simulink model "bai27_Simulink"  (R2016a)
settings: Solver=VariableStepAuto  StartTime=0.0  StopTime=10.0  RelTol=1e-3
settings Model: Creator=HP  LastModifiedBy=HP

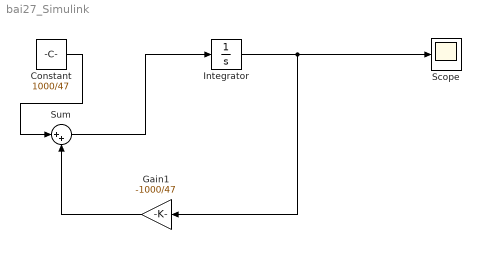
== system bai27_Simulink ==
  Constant : Constant  Value=1000/47
  Gain1 : Gain  Gain=-1000/47
  Integrator : Integrator
  Scope : Scope
  Sum : Sum  Inputs=|++
  wires:
  Integrator/1 -> Gain1/1, Scope/1
  Constant/1 -> Sum/1
  Gain1/1 -> Sum/2
  Sum/1 -> Integrator/1
